simulink model "RL_TTS3_Controller_Blank"  (R2019b)
settings: Solver=FixedStepAuto  StartTime=0.0  StopTime=10.0  FixedStep=0.01  RelTol=1e-3
PostLoadFcn:
  | if any(exist('dsrtsu_mdlpostloadfcn', 'file') ~= 0), dsrtsu_mdlpostloadfcn('Execute', bdroot); end
values from neighbouring files (symbols this model uses):
  Pprev = [15.9081147156 2.96062907929e-12 0.000675171321078 -0.874073498352 4.34237622312e-05 2.96062907929e-12 15.9081147156 0.000675171327952 4.34237625059e-05 -0.874073498351 0.000675171321078 0.000675171327952 ... (25 elements, 5x5)]    [RL_TTS3_Controller_Blank.mat]
  Ts2 = 4    [RL_TTS3_Controller_Blank.mat]
libraries: simulink x1
settings Model: DSRTSU_INTERNAL_RTI_VER=550  DSRTSU_INTERNAL_RTI_TYPE=rti1104  RTICANMMDATA=struct('GeneralSetupData',struct('modelroot','E:\Will\RemoteLabs\TTS3\HostPC','generalsettings',struct('filesettings',struct('destfolder',struct('Name','RTICANMM_FILES','Check',1),'buildfolder',struct('Name','.','Check',1),'AbsDestfolder',struct('Name','E:\Will\RemoteLabs\TTS3\HostPC\RTICANMM_FILES'),'AbsBuildfolder',struct('Name','E:\Will\RemoteLabs\TTS3\HostPC'))),'options',struct('addpaths',1,'rmpaths',1,'addtrcexclusion',true,'cannavigator',struct('checkmonitoring',0),'show_usrtrc',0,'use_usrtrc',0),'advanced',struct('options',ones(1,100)),'MPSetup',{{}},'RTI',struct('Type','RTI1104','Ver','7.13','Date','02-Nov-2019'),'modelname','TTS3_Controller_Test_OL','block','TTS3_Controller_Test_OL'))  DSRTSU_INTERNAL_RTIFPGA=150  Creator=whendrix  LastModifiedBy=maxva
settings OptimizationCC: BlockReduction=off  DefaultParameterBehavior=Inlined  OptimizeBlockIOStorage=off  BufferReuse=off  GlobalBufferReuse=off  ExpressionFolding=off  LocalBlockOutputs=off  OptimizeDataStoreBuffers=off  BusAssignmentInplaceUpdate=off
settings DebuggingCC: BusObjectLabelMismatch=none
settings HardwareCC: ProdBitPerPointer=32  ProdBitPerSizeT=32  ProdBitPerPtrDiffT=32  ProdLargestAtomicInteger=Integer  ProdEndianess=BigEndian  ProdWordSize=32  ProdHWDeviceType=Custom Processor->Custom  TargetIntDivRoundTo=Zero  TargetEndianess=BigEndian  TargetHWDeviceType=Custom Processor->Custom
settings ModelReferenceCC: ModelReferenceNumInstancesAllowed=Single  ModelReferenceMinAlgLoopOccurrences=on
settings SFSimCC: MATLABDynamicMemAlloc=off  CustomCodeUndefinedFunction=UseInterfaceOnly
settings RTWCC: Description=dSPACE DS1104 Hardware Platform  SystemTargetFile=rti1104.tlc  MakeCommand=make_rti  TemplateMakefile=rti1104.tmf
settings CodeAppCC: MaxIdLength=63
settings STFCustomTargetCC: ParMdlRefBuildCompliant=on  SystemTargetFile=rti1104.tlc
settings GRTTargetCC: TargetLangStandard=C89/C90 (ANSI)  CompOptLevelCompliant=off  ConcurrentExecutionCompliant=off  CombineOutputUpdateFcns=off  MatFileLogging=off  CPPClassGenCompliant=off  UseToolchainInfoCompliant=off

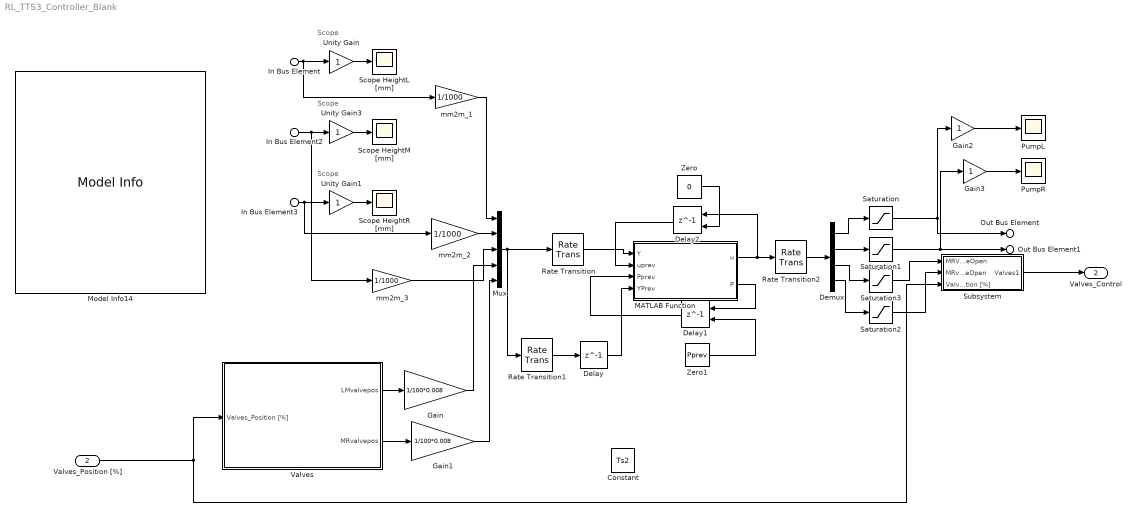
== system RL_TTS3_Controller_Blank ==
  note: Scope
  note: Scope
  note: Scope
  In Bus Element : Inport  PortName=Heights [mm]  Element=Left
  In Bus Element2 : Inport  PortName=Heights [mm]  Element=Middle
  In Bus Element3 : Inport  PortName=Heights [mm]  Element=Right
  Valves_Position [%] : Inport  Port=2  OutDataTypeStr=Bus: ValvesSOCI
  Constant : Constant  Value=Ts2
  Delay : Delay  DelayLength=1
  Delay1 : Delay  DelayLength=1  InitialConditionSource=Input port  SampleTime=Ts2
      settings: InputPortMap=u0,p4
  Delay2 : Delay  DelayLength=1  InitialConditionSource=Input port  SampleTime=Ts2
      settings: InputPortMap=u0,p4
  Demux : Demux
  Gain : Gain  Gain=1/100*0.008
  Gain1 : Gain  Gain=1/100*0.008
  Gain2 : Gain
  Gain3 : Gain
  MATLAB Function : MATLAB Function  TreatAsAtomicUnit=on  SystemSampleTime=Ts2
      settings: MinAlgLoopOccurrences=on
  Model Info14 : simulink/Model-Wide Utilities/Model Info  Frame=on  DisplayStringWithTags=|  HorizontalTextAlignment=Left  LeftAlignmentValue=0.02
      | Start model for the "Three Tank"
      | experiment on the "Three Tank" setup.
      | Version: 1.0
      | 
      | 
      | INFORMATION
      | ----------------------
      | 
      | Unity Gain block before Scope is needed for
      | RemoteLabs compatebility. 
      | Do not modify or remove!
      | 
      | Pump range:
      | 0 to 0.102 [l/s]
      | 
      | The 5 Valves are labeled according 
      | to their position:
      | 
      |    LM  MR
      |      X     X
      |  X      X      X
      | LD    MD   RD
      | 
      | L = Left
      | M = Middle
      | R = Right
      | D = Down
  Mux : Mux  Inputs=5
  PumpL : Scope
  "PumpR " : Scope
  Rate Transition : RateTransition  OutPortSampleTime=Ts2
  Rate Transition1 : RateTransition  OutPortSampleTime=Ts2
  Rate Transition2 : RateTransition  OutPortSampleTime=Ts
  Saturation : Saturate  UpperLimit=0.1  LowerLimit=0
  Saturation1 : Saturate  UpperLimit=0.1  LowerLimit=0
  Saturation2 : Saturate  UpperLimit=100  LowerLimit=0
  Saturation3 : Saturate  UpperLimit=100  LowerLimit=0
  Scope HeightL [mm] : Scope
  Scope HeightM [mm] : Scope
  Scope HeightR [mm] : Scope
  Subsystem : Subsystem
  Unity Gain : Gain
  Unity Gain1 : Gain
  Unity Gain3 : Gain
  Valves : Subsystem  TreatAsAtomicUnit=on
  Zero : Constant  Value=0  OutDataTypeStr=Inherit: Inherit via back propagation
  Zero1 : Constant  Value=Pprev  OutDataTypeStr=Inherit: Inherit via back propagation
  mm2m_1 : Gain  Gain=1/1000
  mm2m_2 : Gain  Gain=1/1000
  mm2m_3 : Gain  Gain=1/1000
  Out Bus Element : Outport  VectorParamsAs1DForOutWhenUnconnected=off  PortName=Pumps [l/s]  Element=Left
  Out Bus Element1 : Outport  VectorParamsAs1DForOutWhenUnconnected=off  PortName=Pumps [l/s]  Element=Right
  Valves_Control : Outport  Port=2  OutDataTypeStr=Bus: ValvesSICO  VectorParamsAs1DForOutWhenUnconnected=off
  wires:
  Unity Gain3/1 -> Scope HeightM [mm]/1
  Unity Gain1/1 -> Scope HeightR [mm]/1
  In Bus Element/1 -> mm2m_1/1, Unity Gain/1
  In Bus Element2/1 -> mm2m_3/1, Unity Gain3/1
  In Bus Element3/1 -> mm2m_2/1, Unity Gain1/1
  Valves_Position [%]/1 -> Valves/1(Valves_Position [%]), Subsystem/3(Valves_Position [%])
  Unity Gain/1 -> Scope HeightL [mm]/1
  MATLAB Function/1(u) -> Delay2/1, Rate Transition2/1
  Demux/1 -> Saturation/1
  Demux/2 -> Saturation1/1
  Mux/1 -> Rate Transition/1, Rate Transition1/1
  Subsystem/1(Valves1) -> Valves_Control/1
  Demux/3 -> Saturation3/1
  Valves/1(LMvalvepos) -> Gain/1
  Gain/1 -> Mux/4
  Valves/2("MRvalvepos ") -> Gain1/1
  Gain1/1 -> Mux/5
  MATLAB Function/2(P) -> Delay1/1
  Delay/1 -> MATLAB Function/4(YPrev)
  Rate Transition/1 -> MATLAB Function/1(Y)
  Rate Transition1/1 -> Delay/1
  Rate Transition2/1 -> Demux/1
  Delay1/1 -> MATLAB Function/3(Pprev)
  Delay2/1 -> MATLAB Function/2(uprev)
  Zero/1 -> Delay2/2
  Zero1/1 -> Delay1/2
  mm2m_1/1 -> Mux/1
  mm2m_2/1 -> Mux/2
  mm2m_3/1 -> Mux/3
  Gain2/1 -> PumpL/1
  Gain3/1 -> "PumpR "/1
  Demux/4 -> Saturation2/1
  Saturation/1 -> Gain2/1, Out Bus Element/1
  Saturation1/1 -> Gain3/1, Out Bus Element1/1
  Saturation2/1 -> Subsystem/2(MRvalveOpen)
  Saturation3/1 -> Subsystem/1("MRValveOpen ")

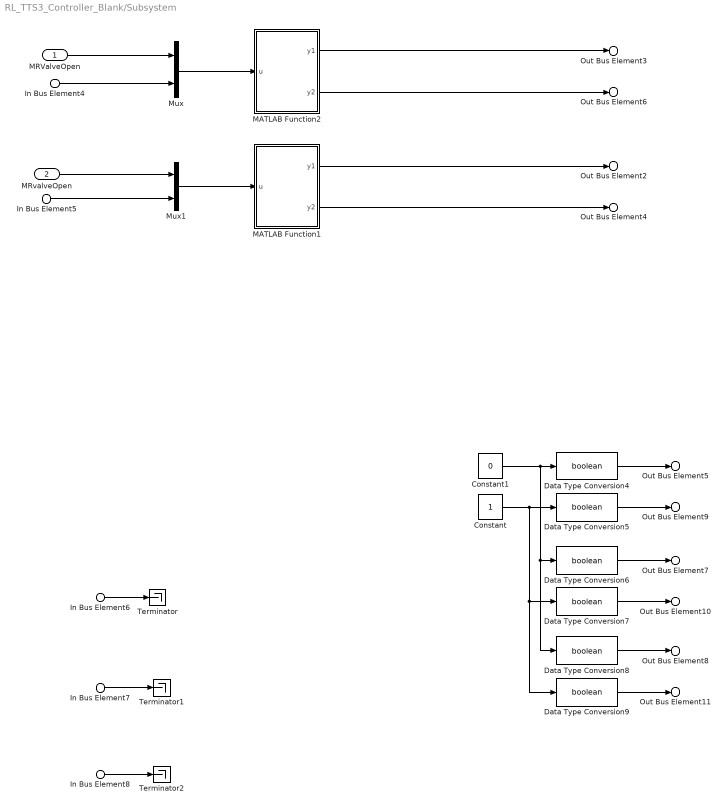
== system RL_TTS3_Controller_Blank/Subsystem ==
  "MRValveOpen " : Inport
  MRvalveOpen : Inport  Port=2
  In Bus Element4 : Inport  Port=3  PortName=Valves_Position [%]  Element=LeftMiddle
  In Bus Element5 : Inport  Port=3  PortName=Valves_Position [%]  Element=MiddleRight
  In Bus Element6 : Inport  Port=3  PortName=Valves_Position [%]  Element=LeftDown
  In Bus Element7 : Inport  Port=3  PortName=Valves_Position [%]  Element=MiddleDown
  In Bus Element8 : Inport  Port=3  PortName=Valves_Position [%]  Element=RightDown
  Constant : Constant
  Constant1 : Constant  Value=0
  Data Type Conversion{4..9} (6 alike) : DataTypeConversion  OutDataTypeStr=boolean
  MATLAB Function1 : MATLAB Function  TreatAsAtomicUnit=on
  MATLAB Function2 : MATLAB Function  TreatAsAtomicUnit=on
  Mux : Mux  Inputs=2
  Mux1 : Mux  Inputs=2
  Terminator : Terminator
  Terminator1 : Terminator
  Terminator2 : Terminator
  Out Bus Element8 : Outport  VectorParamsAs1DForOutWhenUnconnected=off  PortName=Valves1  Element=RightDown.Open
  Out Bus Element11 : Outport  VectorParamsAs1DForOutWhenUnconnected=off  PortName=Valves1  Element=RightDown.Close
  Out Bus Element5 : Outport  VectorParamsAs1DForOutWhenUnconnected=off  PortName=Valves1  Element=LeftDown.Open
  Out Bus Element9 : Outport  VectorParamsAs1DForOutWhenUnconnected=off  PortName=Valves1  Element=LeftDown.Close
  Out Bus Element7 : Outport  VectorParamsAs1DForOutWhenUnconnected=off  PortName=Valves1  Element=MiddleDown.Open
  Out Bus Element10 : Outport  VectorParamsAs1DForOutWhenUnconnected=off  PortName=Valves1  Element=MiddleDown.Close
  Out Bus Element2 : Outport  VectorParamsAs1DForOutWhenUnconnected=off  PortName=Valves1  Element=MiddleRight.Open
  Out Bus Element4 : Outport  VectorParamsAs1DForOutWhenUnconnected=off  PortName=Valves1  Element=MiddleRight.Close
  Out Bus Element3 : Outport  VectorParamsAs1DForOutWhenUnconnected=off  PortName=Valves1  Element=LeftMiddle.Open
  Out Bus Element6 : Outport  VectorParamsAs1DForOutWhenUnconnected=off  PortName=Valves1  Element=LeftMiddle.Close
  wires:
  Data Type Conversion4/1 -> Out Bus Element5/1
  Data Type Conversion5/1 -> Out Bus Element9/1
  Data Type Conversion8/1 -> Out Bus Element8/1
  Constant1/1 -> Data Type Conversion8/1, Data Type Conversion6/1, Data Type Conversion4/1
  Data Type Conversion9/1 -> Out Bus Element11/1
  Data Type Conversion7/1 -> Out Bus Element10/1
  Data Type Conversion6/1 -> Out Bus Element7/1
  Constant/1 -> Data Type Conversion9/1, Data Type Conversion7/1, Data Type Conversion5/1
  In Bus Element6/1 -> Terminator/1
  In Bus Element8/1 -> Terminator2/1
  In Bus Element7/1 -> Terminator1/1
  In Bus Element4/1 -> Mux/2
  Mux/1 -> MATLAB Function2/1(u)
  In Bus Element5/1 -> Mux1/2
  MRvalveOpen/1 -> Mux1/1
  MATLAB Function2/2(y2) -> Out Bus Element6/1
  MATLAB Function2/1(y1) -> Out Bus Element3/1
  "MRValveOpen "/1 -> Mux/1
  Mux1/1 -> MATLAB Function1/1(u)
  MATLAB Function1/1(y1) -> Out Bus Element2/1
  MATLAB Function1/2(y2) -> Out Bus Element4/1

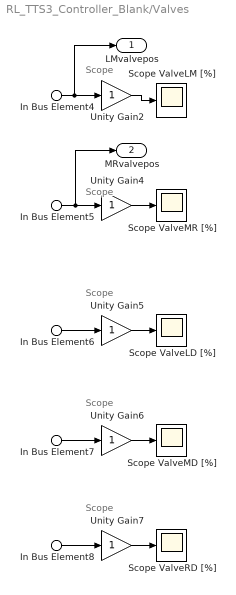
== system RL_TTS3_Controller_Blank/Valves ==
  note: Scope
  note: Scope
  note: Scope
  note: Scope
  note: Scope
  In Bus Element4 : Inport  PortName=Valves_Position [%]  Element=LeftMiddle
  In Bus Element5 : Inport  PortName=Valves_Position [%]  Element=MiddleRight
  In Bus Element6 : Inport  PortName=Valves_Position [%]  Element=LeftDown
  In Bus Element7 : Inport  PortName=Valves_Position [%]  Element=MiddleDown
  In Bus Element8 : Inport  PortName=Valves_Position [%]  Element=RightDown
  Scope ValveLD [%] : Scope
  Scope ValveLM [%] : Scope
  Scope ValveMD [%] : Scope
  Scope ValveMR [%] : Scope
  Scope ValveRD [%] : Scope
  Unity Gain{2,4..7} (5 alike) : Gain
  LMvalvepos : Outport
  "MRvalvepos " : Outport  Port=2
  wires:
  In Bus Element5/1 -> "MRvalvepos "/1, Unity Gain4/1
  In Bus Element4/1 -> Unity Gain2/1, LMvalvepos/1
  In Bus Element7/1 -> Unity Gain6/1
  Unity Gain6/1 -> Scope ValveMD [%]/1
  In Bus Element6/1 -> Unity Gain5/1
  In Bus Element8/1 -> Unity Gain7/1
  Unity Gain7/1 -> Scope ValveRD [%]/1
  Unity Gain4/1 -> Scope ValveMR [%]/1
  Unity Gain5/1 -> Scope ValveLD [%]/1
  Unity Gain2/1 -> Scope ValveLM [%]/1

== matlab function RL_TTS3_Controller_Blank/Subsystem/MATLAB Function2 ==
  data: u input; y1 output; y2 output
function [y1,y2] = fcn(u)
    if abs(u(1)-u(2))<=5
        y1=false;
        y2 = false;
    elseif u(2)>u(1)+5
        y1 = false;
        y2 = true;
    elseif u(1)>u(2)+5
        y1 = true;
        y2 = false;
    else
        y1 = false;
        y2 = false;
    end
end

== matlab function RL_TTS3_Controller_Blank/MATLAB Function ==
  data: Y input; u output; uprev input; Pprev input; YPrev input; P output
function [u, P] = MPC_fcn(Y, uprev, Pprev, YPrev)
% outputs 4d vector u containing inputs for TTS  (format pump1 pump2 valve LM valve RM)
% outputs 3x3 matrix P, containing solution to DARE, can be used in
% next itration
% Y: 5d input state vector of TTS (format water level tank 1, tank 2, tank 3, connecting pipe diameter LM)
% uprev: previous input sent to plant (4D vector, same format as u), for augmented model necessary
% Pprev: previous solution to DARE, might be used if no stabilizing
% solution can be calculated
% Yprev: previous 5d state vector of TTS, same format as Y
%% ini
u = zeros(4,1);
P = zeros(5,5);
%% constants
S = 5e-5;               % [m^2]
Dvalve = sqrt(4*S/pi);     % [m]
Atank = 0.0154;         % [m^2]
g = 9.81;               % [m/s^2]
L = 0.1;                % [m]
mu = 1.002;             % [Ns/m^2]
rho = 1000;             % [kg/m^3]
% system constants (ID or whatever)
v4 = 0.5;                 % [s]?
v5 = 0.5;                 % [s]?

% Constraints 
Hmax = 0.61;            % [m]
Qmax = 0.1;             % [l/s]

% other things
Ts = 1;                 % TODO: check if need be due to .mat file?
N = 5;
%% model
BmCT = [0.001/Atank 0 0 0;
        0 0.001/Atank 0 0;
        0 0 0 0 ;
        0 0 0.01*v4*Dvalve 0;
        0 0 0 0.01*v5*Dvalve];
Cm = eye(5);


m = size(BmCT,2);
n = size(BmCT,1);
q = size(Cm,1);

Dm = zeros(q,m);
%% constraints
deltaumin = [-0.8*Qmax; -0.8*Qmax; -100; -100];
deltaumax = -deltaumin;
umin  = zeros(4,1);
umax  = [Qmax; Qmax; 100; 100];
ymin  = zeros(q,1);
ymax  = [zeros(3,1) + Hmax; Dvalve; Dvalve];

%% reference How to design reference for valves?
r = [zeros(q-2,1)+0.3; zeros(2,1)];
%% Q & R
Q = [eye(3) zeros(3,2);
        zeros(2,5)];
Qm = [  eye(3)      zeros(3,2);
        zeros(2,5)                              ];
R = [eye(2) zeros(2,2);
    zeros(2,2) 0.00001*eye(2)];



% Pprev = [15.9081147155710,2.96062907928527e-12,0.000675171321078397,-0.874073498351786,4.34237622311551e-05;2.96062907928527e-12,15.9081147155711,0.000675171327952177,4.34237625058848e-05,-0.874073498351258;0.000675171321078397,0.000675171327952177,155486.683787255,9999.99731184461,9999.99731184459;-0.874073498351786,4.34237625058848e-05,9999.99731184461,643.201217531435,643.148089872505;4.34237622311551e-05,-0.874073498351258,9999.99731184459,643.148089872505,643.201217531434];
P = Pprev;
% Omega
Phi = zeros(N*n,2*n);
Gamma = zeros(N*n,N*m);

Psi = zeros(m*N,m*N);
Omega = zeros(n*N,n*N);
for Pi = 1:N
    Psi((Pi-1)*m+1:Pi*m,(Pi-1)*m+1:Pi*m) = R;
end

for oi = 1:N-1
    Omega((oi-1)*n+1:oi*n,(oi-1)*n+1:oi*n) = Q;
end
Omega(end-n+1:end,end-n+1:end) = P;


AmCT = freeFallLinearizationA(Y);
Dmatrix = expm([AmCT BmCT;zeros(m,m+n)]*Ts);
Am = Dmatrix(1:n,1:n);
Bm = Dmatrix(1:n,n+1:end);


A = [Am zeros(q,n)';
     Cm*Am eye(q)];
B = [Bm;Cm*Bm];
C = [zeros(q,n) eye(q)];
Xaug = zeros(2*q,1);
Xaug = [    Y-YPrev;
            Y           ];




mphi = 4;
qphi = 5;
for i = 1:N
   Phi((i-1)*qphi+1:i*qphi,:) = C*A^i;
end

for i = 1:N
    for j = 1:i
        Gamma((i-1)*qphi+1:qphi*i,(j-1)*mphi+1:j*mphi) = C*A^(i-j)*B;
    end
end


G = 2*(Psi+Gamma'*Omega*Gamma);
F = 2*Gamma'*Omega;

Rk = zeros(N*5,1);
for ii = 1:N
    Rk((ii-1)*5+1:ii*5) = r;
end

[D,M,E,c] = DMEcIntegral(deltaumin,deltaumax,umin,umax,ymin,ymax,uprev,N);


Lmpc = M*Gamma+E;
W = -D*C-M*Phi;
u_qp = zeros(N*m,1);
invH = inv((G+G')/2);
[u_qp] = HildrethSolver_Vanilla((G+G')/2,(F*Phi*Xaug-F*Rk),Lmpc,c+W*Xaug,20000,1,deltaumin,deltaumax);

deltaustar0k = zeros(m,1);
deltaustar0k = [eye(m) zeros(m,m*(N-1))]*u_qp;
u = uprev + deltaustar0k;
%%-------------------------------------------------------------------------
% functions
function A = freeFallLinearizationA(x)
tol = 0;
if ((x(2)-x(3)) <= tol) && ((x(1)-x(3)) > tol)
    A = [   
        -S*x(4)/Dvalve*g/sqrt(2*g*abs(x(1)-x(3)))/Atank    0    S*x(4)/Dvalve*g/sqrt(2*g*abs(x(1)-x(3)))/Atank     -sign(x(1)-x(3))*S/Dvalve*sqrt(2*g*abs(x(1)-x(3)))/Atank   0;
        zeros(1,5);
        S*x(4)/Dvalve*g/sqrt(2*g*abs(x(1)-x(3)))/Atank     0    -S*x(4)/Dvalve*g/sqrt(2*g*abs(x(1)-x(3)))/Atank    sign(x(1)-x(3))*S/Dvalve*sqrt(2*g*abs(x(1)-x(3)))/Atank    0;
        0                       0                       0                                   -v4                                     0;
        0                       0                       0                                   0                                       -v5
        ];
elseif ((x(1)-x(3)) <= tol) && ((x(2)-x(3)) > tol)
    A = [   
        zeros(1,5);
        0                       -S*x(5)/Dvalve*g/sqrt(2*g*abs(x(2)-x(3)))/Atank    S*x(5)/Dvalve*g/sqrt(2*g*abs(x(2)-x(3)))/Atank     0    -sign(x(2)-x(3))*S/Dvalve*sqrt(2*g*abs(x(2)-x(3)))/Atank;
        0                       S*x(5)/Dvalve*g/sqrt(2*g*abs(x(2)-x(3)))/Atank     -S*x(5)/Dvalve*g/sqrt(2*g*abs(x(2)-x(3)))/Atank    0    sign(x(2)-x(3))*S/Dvalve*sqrt(2*g*abs(x(2)-x(3)))/Atank;
        0                       0                       0                                   -v4                                     0;
        0                       0                       0                                   0                                       -v5
        ];
elseif ((x(2)-x(3)) <= tol) && ((x(1)-x(3)) <= tol)
     A = [   
        zeros(3,5);
        0                       0                       0                                   -v4                                     0;
        0                       0                       0                                   0                                       -v5
        ];
else
    A = [   
        -S*x(4)/Dvalve*g/sqrt(2*g*abs(x(1)-x(3)))/Atank     0                                                   sign(x(1)-x(3))*S*x(4)/Dvalve*g/sqrt(2*g*abs(x(1)-x(3)))/Atank                                                      -S/Dvalve*sqrt(2*g*abs(x(1)-x(3)))/Atank   0;
        0                                                   -S*x(5)/Dvalve*g/sqrt(2*g*abs(x(2)-x(3)))/Atank     sign(x(2)-x(3))*S*x(5)/Dvalve*g/sqrt(2*g*abs(x(2)-x(3)))/Atank                                                      0                                       -S/Dvalve*sqrt(2*g*abs(x(2)-x(3)))/Atank;
        S*x(4)/Dvalve*g/sqrt(2*g*abs(x(1)-x(3)))/Atank      S*x(5)/Dvalve*g/sqrt(2*g*abs(x(2)-x(3)))/Atank      -sign(x(1)-x(3))*S*x(4)/Dvalve*g/sqrt(2*g*abs(x(1)-x(3)))/Atank-sign(x(2)-x(3))*S*x(5)/Dvalve*g/sqrt(2*g*abs(x(2)-x(3)))/Atank      S/Dvalve*sqrt(2*g*abs(x(1)-x(3)))/Atank    S/Dvalve*sqrt(2*g*abs(x(2)-x(3)))/Atank;
        0                       0                       0                                   -v4                                     0;
        0                       0                       0                                   0                                       -v5
        ];
end
end

%%-------------------------------------------------------------------------
function [D,M,E,c] = DMEcIntegral(deltaumin,deltaumax,umin,umax,ymin,ymax,ukmin1,N)
mDMEC = size(umin,1);
qDMEC = size(ymin,1);

bi = [-deltaumin; deltaumax; -umin+ukmin1;umax-ukmin1;-ymin;ymax];
bN = [zeros(4*mDMEC,1);-ymin; ymax];
Lb = length(bi);

c = zeros((4*mDMEC+2*qDMEC)*(N+1),1);
for i = 1:N
    c((i-1)*Lb+1:i*Lb) = bi;
end
c(N*Lb+1:end,:) = bN;


M0 = [zeros(4*mDMEC,qDMEC); -eye(qDMEC); eye(qDMEC)];

D = zeros((4*mDMEC+2*qDMEC)*(N+1),qDMEC);
D(1:size(M0,1),:)  = M0;

M = zeros((4*mDMEC+2*qDMEC)*(N+1),qDMEC*N);
for i = 1:N
    M(i*Lb+1:(i+1)*Lb,(i-1)*qDMEC+1:i*qDMEC) = M0;
end

Ei = [-eye(mDMEC); eye(mDMEC);-eye(mDMEC); eye(mDMEC);zeros(2*qDMEC,mDMEC)];
E0ff = [zeros(2*mDMEC,mDMEC);-eye(mDMEC); eye(mDMEC);zeros(2*qDMEC,mDMEC)];

E = zeros((4*mDMEC+2*qDMEC)*(N+1),mDMEC*N);
for i = 1:N
    E((i-1)*Lb+1:(i)*Lb,(i-1)*mDMEC+1:i*mDMEC) = Ei;
    if i > 1
        for j = 1:i-1
            E((i-1)*Lb+1:(i)*Lb,(j-1)*mDMEC+1:j*mDMEC) = E0ff;
        end
    end
end

end
%--------------------------------------------------------------------------
function [U_k] = HildrethSolver_Vanilla(G,F,L,cplusWxk,MaxIter,ErrorBound,umin,umax)
% this is our vanilla Hildreth solver and this script has some differnt varianames, but is for the rest identical
% The equation (1/2)u'Gu+u'F, s.t. Lu <= cplusWxk is optimized

% calculate unconstraint solution first
U_k_unconstraint = -G\(F);

if(any(L*U_k_unconstraint>cplusWxk))
    % constraints violated
    H = L*(G\transpose(L));
    K = cplusWxk + L*(G\(F));
    % now ideally -H*lambdastar=K, but often not invertible
    nH = size(H,1); % nr of lambdas to solve
    lambdas = zeros(nH,1);
    mHi=1; % iteration counter
    
    while(1)
        % update for next interation
        lambdas_old = lambdas;
        
        % update each scalar value
        for i = 1:nH
            lambdas(i,1) = max(0,-(K(i) + H(i,:)*lambdas - H(i,i)*lambdas(i,1))/H(i,i));
        end     
        % if maximum is reached without finding a feasible solution
        if(mHi>MaxIter)
           fprintf('No feasible solution found within nr. of iterations.\n');
           U_k = U_k_unconstraint;
           for i = 1:length(umin)
            if U_k(i:4:end) < umin(i)
                U_k(i:4:end) = umin(i);
            elseif U_k(i:4:end) > umax(i)
                U_k(i:4:end) = umax(i);
            end
           end
           
           
           return;
%            break
        end
        % check for convergence or timelimit
        if(transpose(lambdas-lambdas_old)*(lambdas-lambdas_old)<=ErrorBound)
            break
        end
        
        % update nr of iterations
        mHi = mHi+1;
    end
    
    % calculate optimal input
    U_k = -G\(F+transpose(L)*lambdas);
else
    % constraints not violated
    U_k = U_k_unconstraint;
%     lambdas = zeros(size(L,1),1);
end
end
end

== matlab function RL_TTS3_Controller_Blank/Subsystem/MATLAB Function1 ==
  data: u input; y1 output; y2 output
function [y1,y2] = fcn(u)
    if abs(u(1)-u(2))<=5
        y1=false;
        y2 = false;
    elseif u(2)>u(1)+5
        y1 = false;
        y2 = true;
    elseif u(1)>u(2)+5
        y1 = true;
        y2 = false;
    else
        y1 = false;
        y2 = false;
    end
end
